simulink model "functionLookupTable"  (R2023b)
settings: Solver=VariableStepAuto  StartTime=0.0  StopTime=10.0  RelTol=1e-3
settings Model: Creator=NITRO  LastModifiedBy=NITRO

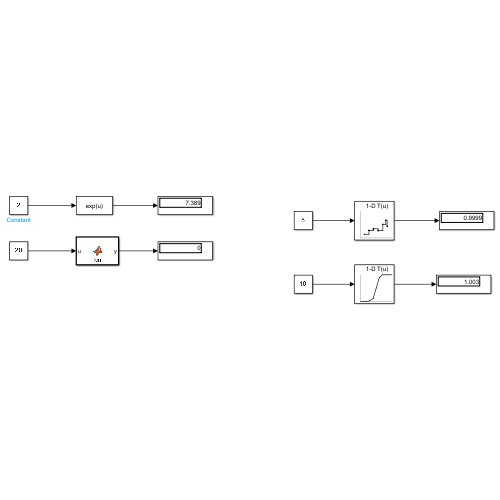
[thumbnail: Simulink's stored preview of the top-level diagram]
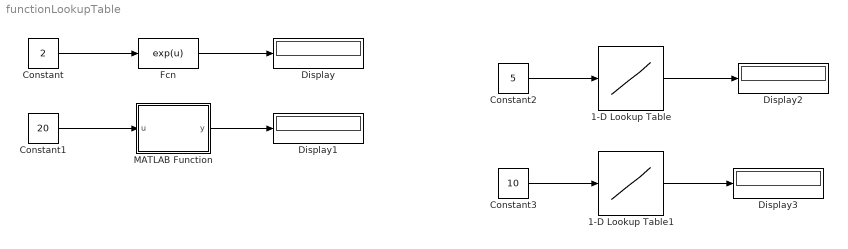
== system functionLookupTable ==
  1-D Lookup Table : Lookup_n-D  NumberOfTableDimensions=1  LookupTableObject=''  BreakpointsForDimension1=[-5:5]  BreakpointsForDimension1FirstPoint=10  BreakpointsForDimension2FirstPoint=10  BreakpointsForDimension1Spacing=12  BreakpointsForDimension2Spacing=12  IndexSearchMethod=Evenly spaced points  Table=tanh([-5:5])  InterpMethod=Flat  DiagnosticForOutOfRangeInput=Error  InternalRulePriority=Speed  RndMeth=Simplest
  1-D Lookup Table1 : Lookup_n-D  NumberOfTableDimensions=1  BreakpointsForDimension1=[-5:5]  Table=tanh([-5:5])  InternalRulePriority=Speed  RndMeth=Simplest
  Constant : Constant  Value=2
  Constant1 : Constant  Value=20
  Constant2 : Constant  Value=5
  Constant3 : Constant  Value=10
  Display{,1..3} (4 alike) : Display
  Fcn : Fcn  Expr=exp(u)
  MATLAB Function : MATLAB Function  TreatAsAtomicUnit=on
  wires:
  Constant/1 -> Fcn/1
  Fcn/1 -> Display/1
  Constant1/1 -> MATLAB Function/1(u)
  MATLAB Function/1(y) -> Display1/1
  Constant2/1 -> 1-D Lookup Table/1
  1-D Lookup Table/1 -> Display2/1
  1-D Lookup Table1/1 -> Display3/1
  Constant3/1 -> 1-D Lookup Table1/1

== matlab function functionLookupTable/MATLAB Function ==
  data: u input; y output
function y = fcn(u)

if u>= 25
    y = 1;
else
    y = 0;

end
